simulink model "SensorFaultInj"  (R2013a)
settings: Solver=FixedStepDiscrete  SolverMode=SingleTasking  StartTime=0.0  StopTime=SimLength  FixedStep=SampleTime  RelTol=1e-3
values from neighbouring files (symbols this model uses):
  GlobalSeed = 10    [start_framework07.m]
  SampleTime = 0.01    [start_framework07.m]
  SimLength = 40    [start_framework07.m]
undefined symbols (not defined in the file or in its folder): DiscIntNeverNeededParam
libraries: dspswit3 x48, simulink x32
(part 6 of 9)

== system SensorFaultInj/FIM_Muster2/Parser Modul/schedule once per sample step /schedule_fcn id 6 ==
  In1 : Inport
  Discrete-Time Integrator : DiscreteIntegrator  SampleTime=-1  ICPrevOutput=DiscIntNeverNeededParam  ICPrevScaledInput=DiscIntNeverNeededParam
  Scope1 : Scope  NumInputPorts=2
      settings: YMin=-5~-5  YMax=5~5  SaveName=ScopeData25
  SimLength : Constant  Value=SimLength
  ex_sfun_schedulefcn1 : S-Function  FunctionName=ex_sfun_schedulefcn  EnableBusSupport=off  mask(Legacy Function){SFunctionSpec=single y1 = schedule_fcn(double u1, double u2, single u3, single u4), ShowSpec=on}
      mask prompts: ShowSpec "Display function specification"
      mask help:
      | This block allows you to call the legacy functions specified by the following Legacy Code Tool definition:
      | def.SFunctionName = 'ex_sfun_schedulefcn';
      | def.OutputFcnSpec = 'single y1 = schedule_fcn(double u1, double u2, single u3, single u4)';
      | def.HeaderFiles = {'schedule_fcn.hpp'};
      | def.SourceFiles = {'schedule_fcn.cpp'};
      | def.Options.language = 'C++';
      mask Help: <p>This block was generated automatically by the Legacy Code Tool. For detailed help on this tool, call<a href="matlab:legacy_code('help')"> legacy_code('help')</a>.</p>
      mask Callback ShowSpec:
      | if strcmp(get_param(gcbh, 'ShowSpec'), 'on')
      |   set_param(gcbh, 'MaskDisplay', sprintf('fprintf(''%s'');', get_param(gcbh, 'SFunctionSpec')));
      | else
      |   set_param(gcbh, 'MaskDisplay', sprintf('fprintf(''%s'');', get_param(gcbh, 'FunctionName')));
      | end
      mask Display: fprintf('single y1 = schedule_fcn(double u1, double u2, single u3, single u4)');
  "fault_id " : Constant  Value=6  OutDataTypeStr=single
  one : Constant
  output : Outport  OutputWhenDisabled=reset  InitialOutput=[0]
  wires:
  one/1 -> Discrete-Time Integrator/1
  Discrete-Time Integrator/1 -> ex_sfun_schedulefcn1/2, Scope1/2
  ex_sfun_schedulefcn1/1 -> Scope1/1, output/1  "out_schedule"
  SimLength/1 -> ex_sfun_schedulefcn1/1
  "fault_id "/1 -> ex_sfun_schedulefcn1/3
  In1/1 -> ex_sfun_schedulefcn1/4

== system SensorFaultInj/FIM_Muster2/Parser Modul/schedule once per sample step /schedule_fcn id 7 ==
  In1 : Inport
  Discrete-Time Integrator : DiscreteIntegrator  SampleTime=-1  ICPrevOutput=DiscIntNeverNeededParam  ICPrevScaledInput=DiscIntNeverNeededParam
  Scope1 : Scope  NumInputPorts=2
      settings: YMin=-5~-5  YMax=5~5  SaveName=ScopeData25
  SimLength : Constant  Value=SimLength
  ex_sfun_schedulefcn1 : S-Function  FunctionName=ex_sfun_schedulefcn  EnableBusSupport=off  mask(Legacy Function){SFunctionSpec=single y1 = schedule_fcn(double u1, double u2, single u3, single u4), ShowSpec=on}
      mask prompts: ShowSpec "Display function specification"
      mask help:
      | This block allows you to call the legacy functions specified by the following Legacy Code Tool definition:
      | def.SFunctionName = 'ex_sfun_schedulefcn';
      | def.OutputFcnSpec = 'single y1 = schedule_fcn(double u1, double u2, single u3, single u4)';
      | def.HeaderFiles = {'schedule_fcn.hpp'};
      | def.SourceFiles = {'schedule_fcn.cpp'};
      | def.Options.language = 'C++';
      mask Help: <p>This block was generated automatically by the Legacy Code Tool. For detailed help on this tool, call<a href="matlab:legacy_code('help')"> legacy_code('help')</a>.</p>
      mask Callback ShowSpec:
      | if strcmp(get_param(gcbh, 'ShowSpec'), 'on')
      |   set_param(gcbh, 'MaskDisplay', sprintf('fprintf(''%s'');', get_param(gcbh, 'SFunctionSpec')));
      | else
      |   set_param(gcbh, 'MaskDisplay', sprintf('fprintf(''%s'');', get_param(gcbh, 'FunctionName')));
      | end
      mask Display: fprintf('single y1 = schedule_fcn(double u1, double u2, single u3, single u4)');
  "fault_id " : Constant  Value=7  OutDataTypeStr=single
  one : Constant
  output : Outport  OutputWhenDisabled=reset  InitialOutput=[0]
  wires:
  one/1 -> Discrete-Time Integrator/1
  Discrete-Time Integrator/1 -> ex_sfun_schedulefcn1/2, Scope1/2
  ex_sfun_schedulefcn1/1 -> Scope1/1, output/1  "spi_schedule"
  SimLength/1 -> ex_sfun_schedulefcn1/1
  "fault_id "/1 -> ex_sfun_schedulefcn1/3
  In1/1 -> ex_sfun_schedulefcn1/4

== system SensorFaultInj/FIM_Muster2/Parser Modul/schedule once per sample step /schedule_fcn id 8 ==
  In1 : Inport
  Discrete-Time Integrator : DiscreteIntegrator  SampleTime=-1  ICPrevOutput=DiscIntNeverNeededParam  ICPrevScaledInput=DiscIntNeverNeededParam
  Scope1 : Scope  NumInputPorts=2
      settings: YMin=-5~-5  YMax=5~5  SaveName=ScopeData25
  SimLength : Constant  Value=SimLength
  ex_sfun_schedulefcn1 : S-Function  FunctionName=ex_sfun_schedulefcn  EnableBusSupport=off  mask(Legacy Function){SFunctionSpec=single y1 = schedule_fcn(double u1, double u2, single u3, single u4), ShowSpec=on}
      mask prompts: ShowSpec "Display function specification"
      mask help:
      | This block allows you to call the legacy functions specified by the following Legacy Code Tool definition:
      | def.SFunctionName = 'ex_sfun_schedulefcn';
      | def.OutputFcnSpec = 'single y1 = schedule_fcn(double u1, double u2, single u3, single u4)';
      | def.HeaderFiles = {'schedule_fcn.hpp'};
      | def.SourceFiles = {'schedule_fcn.cpp'};
      | def.Options.language = 'C++';
      mask Help: <p>This block was generated automatically by the Legacy Code Tool. For detailed help on this tool, call<a href="matlab:legacy_code('help')"> legacy_code('help')</a>.</p>
      mask Callback ShowSpec:
      | if strcmp(get_param(gcbh, 'ShowSpec'), 'on')
      |   set_param(gcbh, 'MaskDisplay', sprintf('fprintf(''%s'');', get_param(gcbh, 'SFunctionSpec')));
      | else
      |   set_param(gcbh, 'MaskDisplay', sprintf('fprintf(''%s'');', get_param(gcbh, 'FunctionName')));
      | end
      mask Display: fprintf('single y1 = schedule_fcn(double u1, double u2, single u3, single u4)');
  "fault_id " : Constant  Value=8  OutDataTypeStr=single
  one : Constant
  output : Outport  OutputWhenDisabled=reset  InitialOutput=[0]
  wires:
  one/1 -> Discrete-Time Integrator/1
  Discrete-Time Integrator/1 -> ex_sfun_schedulefcn1/2, Scope1/2
  ex_sfun_schedulefcn1/1 -> Scope1/1, output/1  "stz_schedule"
  SimLength/1 -> ex_sfun_schedulefcn1/1
  "fault_id "/1 -> ex_sfun_schedulefcn1/3
  In1/1 -> ex_sfun_schedulefcn1/4

== system SensorFaultInj/FIM_Muster2/Parser Modul/schedule once per sample step /schedule_fcn id 9 ==
  In1 : Inport
  Discrete-Time Integrator : DiscreteIntegrator  SampleTime=-1  ICPrevOutput=DiscIntNeverNeededParam  ICPrevScaledInput=DiscIntNeverNeededParam
  Scope1 : Scope  NumInputPorts=2
      settings: YMin=-5~-5  YMax=5~5  SaveName=ScopeData25
  SimLength : Constant  Value=SimLength
  ex_sfun_schedulefcn1 : S-Function  FunctionName=ex_sfun_schedulefcn  EnableBusSupport=off  mask(Legacy Function){SFunctionSpec=single y1 = schedule_fcn(double u1, double u2, single u3, single u4), ShowSpec=on}
      mask prompts: ShowSpec "Display function specification"
      mask help:
      | This block allows you to call the legacy functions specified by the following Legacy Code Tool definition:
      | def.SFunctionName = 'ex_sfun_schedulefcn';
      | def.OutputFcnSpec = 'single y1 = schedule_fcn(double u1, double u2, single u3, single u4)';
      | def.HeaderFiles = {'schedule_fcn.hpp'};
      | def.SourceFiles = {'schedule_fcn.cpp'};
      | def.Options.language = 'C++';
      mask Help: <p>This block was generated automatically by the Legacy Code Tool. For detailed help on this tool, call<a href="matlab:legacy_code('help')"> legacy_code('help')</a>.</p>
      mask Callback ShowSpec:
      | if strcmp(get_param(gcbh, 'ShowSpec'), 'on')
      |   set_param(gcbh, 'MaskDisplay', sprintf('fprintf(''%s'');', get_param(gcbh, 'SFunctionSpec')));
      | else
      |   set_param(gcbh, 'MaskDisplay', sprintf('fprintf(''%s'');', get_param(gcbh, 'FunctionName')));
      | end
      mask Display: fprintf('single y1 = schedule_fcn(double u1, double u2, single u3, single u4)');
  "fault_id " : Constant  Value=9  OutDataTypeStr=single
  one : Constant
  output : Outport  OutputWhenDisabled=reset  InitialOutput=[0]
  wires:
  one/1 -> Discrete-Time Integrator/1
  Discrete-Time Integrator/1 -> ex_sfun_schedulefcn1/2, Scope1/2
  ex_sfun_schedulefcn1/1 -> Scope1/1, output/1  "stx_schedule"
  SimLength/1 -> ex_sfun_schedulefcn1/1
  "fault_id "/1 -> ex_sfun_schedulefcn1/3
  In1/1 -> ex_sfun_schedulefcn1/4

== system SensorFaultInj/FIM_Muster/Fault Injection Modul/AFI - additive faults injection/non correated noise/pdf_parser ==
  xml id : Inport
  Constant : Constant
  Interpreted MATLAB Function : MATLABFcn  MATLABFcn=rand
  Scope : Scope  NumInputPorts=2
      settings: YMin=0~2.77556e-17  YMax=1~1  SaveName=ScopeData26  MaxDataPoints=50000
  ex_sfun_parsdistr : S-Function  FunctionName=ex_sfun_parsdistr  EnableBusSupport=off  mask(Legacy Function){SFunctionSpec=double y1 = pars_distr(single u1, single u2, double u3), ShowSpec=on}
      mask prompts: ShowSpec "Display function specification"
      mask help:
      | This block allows you to call the legacy functions specified by the following Legacy Code Tool definition:
      | def.SFunctionName = 'ex_sfun_parsdistr';
      | def.OutputFcnSpec = 'double y1 = pars_distr(single u1, single u2, double u3)';
      | def.HeaderFiles = {'pars_distr.hpp'};
      | def.SourceFiles = {'pars_distr.cpp'};
      | def.Options.language = 'C++';
      mask Help: <p>This block was generated automatically by the Legacy Code Tool. For detailed help on this tool, call<a href="matlab:legacy_code('help')"> legacy_code('help')</a>.</p>
      mask Callback ShowSpec:
      | if strcmp(get_param(gcbh, 'ShowSpec'), 'on')
      |   set_param(gcbh, 'MaskDisplay', sprintf('fprintf(''%s'');', get_param(gcbh, 'SFunctionSpec')));
      | else
      |   set_param(gcbh, 'MaskDisplay', sprintf('fprintf(''%s'');', get_param(gcbh, 'FunctionName')));
      | end
      mask Display: fprintf('double y1 = pars_distr(single u1, single u2, double u3)');
  "fault_id " : Constant  Value=5  OutDataTypeStr=single
  distr value : Outport
  wires:
  "fault_id "/1 -> ex_sfun_parsdistr/1
  xml id/1 -> ex_sfun_parsdistr/2
  ex_sfun_parsdistr/1 -> Scope/1, distr value/1
  Constant/1 -> Interpreted MATLAB Function/1
  Interpreted MATLAB Function/1 -> ex_sfun_parsdistr/3, Scope/2

== system SensorFaultInj/FIM_Muster/Fault Injection Modul/AFI - additive faults injection/stuck at x generation/Triggered Subsystem1 ==
  "In1 " : Inport
  Trigger : TriggerPort  TriggerType=either  PortDimensions=1
  Out1 : Outport
  wires:
  "In1 "/1 -> Out1/1

== system SensorFaultInj/FIM_Muster/Fault Injection Modul/AFI - additive faults injection/stuck at x generation1/Triggered Subsystem ==
  top border : Inport
  bottom border : Inport  Port=2
  Trigger : TriggerPort  TriggerType=either  PortDimensions=1
  Add1 : Sum
  Product2 : Product
  Scope : Scope
      settings: YMin=3  YMax=13  SaveName=ScopeData5
  Subtract : Sum  Inputs=+-
  Uniform Random Number : UniformRandomNumber  Minimum=0
  Out1 : Outport
  wires:
  Uniform Random Number/1 -> Product2/2
  top border/1 -> Subtract/1
  Subtract/1 -> Product2/1
  Product2/1 -> Add1/1
  Add1/1 -> Out1/1, Scope/1
  bottom border/1 -> Add1/2, Subtract/2

== system SensorFaultInj/FIM_Muster/Fault Injection Modul/FFI - functional fault injection/time correlated delay /expr_parser ==
  xml id : Inport
  Discrete-Time Integrator : DiscreteIntegrator  SampleTime=-1  ICPrevOutput=DiscIntNeverNeededParam  ICPrevScaledInput=DiscIntNeverNeededParam
  SampleTime : Constant  Value=SampleTime
  Scope1 : Scope  NumInputPorts=2
      settings: YMin=-5~-5  YMax=5~5  SaveName=ScopeData24
  SimLength : Constant  Value=SimLength
  ex_sfun_parsfcn : S-Function  FunctionName=ex_sfun_parsfcn  EnableBusSupport=off  mask(Legacy Function){SFunctionSpec=double y1 = pars_fcn(double u1, double u2, double u3, double u4, single u5), ShowSpec=on}
      mask prompts: ShowSpec "Display function specification"
      mask help:
      | This block allows you to call the legacy functions specified by the following Legacy Code Tool definition:
      | def.SFunctionName = 'ex_sfun_parsfcn';
      | def.OutputFcnSpec = 'double y1 = pars_fcn(double u1, double u2, double u3, double u4, single u5)';
      | def.HeaderFiles = {'pars_fcn.hpp'};
      | def.SourceFiles = {'pars_fcn.cpp'};
      | def.Options.language = 'C++';
      mask Help: <p>This block was generated automatically by the Legacy Code Tool. For detailed help on this tool, call<a href="matlab:legacy_code('help')"> legacy_code('help')</a>.</p>
      mask Callback ShowSpec:
      | if strcmp(get_param(gcbh, 'ShowSpec'), 'on')
      |   set_param(gcbh, 'MaskDisplay', sprintf('fprintf(''%s'');', get_param(gcbh, 'SFunctionSpec')));
      | else
      |   set_param(gcbh, 'MaskDisplay', sprintf('fprintf(''%s'');', get_param(gcbh, 'FunctionName')));
      | end
      mask Display: fprintf('double y1 = pars_fcn(double u1, double u2, double u3, double u4, single u5)');
  "fault_id " : Constant  Value=3
  one : Constant
  corelation value : Outport
  wires:
  one/1 -> Discrete-Time Integrator/1
  Discrete-Time Integrator/1 -> ex_sfun_parsfcn/4, Scope1/2
  "fault_id "/1 -> ex_sfun_parsfcn/1
  SampleTime/1 -> ex_sfun_parsfcn/2
  SimLength/1 -> ex_sfun_parsfcn/3
  xml id/1 -> ex_sfun_parsfcn/5
  ex_sfun_parsfcn/1 -> Scope1/1, corelation value/1

== system SensorFaultInj/FIM_Muster/Fault Injection Modul/MFI - multiplicative fault injection/time correlated noise/expr_parser1 ==
  xml id : Inport
  Discrete-Time Integrator : DiscreteIntegrator  SampleTime=-1  ICPrevOutput=DiscIntNeverNeededParam  ICPrevScaledInput=DiscIntNeverNeededParam
  SampleTime : Constant  Value=SampleTime
  Scope1 : Scope  NumInputPorts=2
      settings: YMin=-5~-5  YMax=5~5  SaveName=ScopeData24
  SimLength : Constant  Value=SimLength
  ex_sfun_parsfcn : S-Function  FunctionName=ex_sfun_parsfcn  EnableBusSupport=off  mask(Legacy Function){SFunctionSpec=double y1 = pars_fcn(double u1, double u2, double u3, double u4, single u5), ShowSpec=on}
      mask prompts: ShowSpec "Display function specification"
      mask help:
      | This block allows you to call the legacy functions specified by the following Legacy Code Tool definition:
      | def.SFunctionName = 'ex_sfun_parsfcn';
      | def.OutputFcnSpec = 'double y1 = pars_fcn(double u1, double u2, double u3, double u4, single u5)';
      | def.HeaderFiles = {'pars_fcn.hpp'};
      | def.SourceFiles = {'pars_fcn.cpp'};
      | def.Options.language = 'C++';
      mask Help: <p>This block was generated automatically by the Legacy Code Tool. For detailed help on this tool, call<a href="matlab:legacy_code('help')"> legacy_code('help')</a>.</p>
      mask Callback ShowSpec:
      | if strcmp(get_param(gcbh, 'ShowSpec'), 'on')
      |   set_param(gcbh, 'MaskDisplay', sprintf('fprintf(''%s'');', get_param(gcbh, 'SFunctionSpec')));
      | else
      |   set_param(gcbh, 'MaskDisplay', sprintf('fprintf(''%s'');', get_param(gcbh, 'FunctionName')));
      | end
      mask Display: fprintf('double y1 = pars_fcn(double u1, double u2, double u3, double u4, single u5)');
  "fault_id " : Constant  Value=2
  one : Constant
  corelation value : Outport
  wires:
  one/1 -> Discrete-Time Integrator/1
  Discrete-Time Integrator/1 -> ex_sfun_parsfcn/4, Scope1/2
  "fault_id "/1 -> ex_sfun_parsfcn/1
  SampleTime/1 -> ex_sfun_parsfcn/2
  SimLength/1 -> ex_sfun_parsfcn/3
  xml id/1 -> ex_sfun_parsfcn/5
  ex_sfun_parsfcn/1 -> Scope1/1, corelation value/1

== system SensorFaultInj/FIM_Muster/Fault Injection Modul/MFI - multiplicative fault injection/time correlated noise/pdf_parser ==
  xml id : Inport
  Constant : Constant
  Interpreted MATLAB Function : MATLABFcn  MATLABFcn=rand
  Scope : Scope  NumInputPorts=2
      settings: YMin=0.05~2.77556e-17  YMax=0.85~1  SaveName=ScopeData26  MaxDataPoints=50000
  ex_sfun_parsdistr : S-Function  FunctionName=ex_sfun_parsdistr  EnableBusSupport=off  mask(Legacy Function){SFunctionSpec=double y1 = pars_distr(single u1, single u2, double u3), ShowSpec=on}
      mask prompts: ShowSpec "Display function specification"
      mask help:
      | This block allows you to call the legacy functions specified by the following Legacy Code Tool definition:
      | def.SFunctionName = 'ex_sfun_parsdistr';
      | def.OutputFcnSpec = 'double y1 = pars_distr(single u1, single u2, double u3)';
      | def.HeaderFiles = {'pars_distr.hpp'};
      | def.SourceFiles = {'pars_distr.cpp'};
      | def.Options.language = 'C++';
      mask Help: <p>This block was generated automatically by the Legacy Code Tool. For detailed help on this tool, call<a href="matlab:legacy_code('help')"> legacy_code('help')</a>.</p>
      mask Callback ShowSpec:
      | if strcmp(get_param(gcbh, 'ShowSpec'), 'on')
      |   set_param(gcbh, 'MaskDisplay', sprintf('fprintf(''%s'');', get_param(gcbh, 'SFunctionSpec')));
      | else
      |   set_param(gcbh, 'MaskDisplay', sprintf('fprintf(''%s'');', get_param(gcbh, 'FunctionName')));
      | end
      mask Display: fprintf('double y1 = pars_distr(single u1, single u2, double u3)');
  "fault_id " : Constant  Value=3  OutDataTypeStr=single
  distr value : Outport
  wires:
  "fault_id "/1 -> ex_sfun_parsdistr/1
  xml id/1 -> ex_sfun_parsdistr/2
  ex_sfun_parsdistr/1 -> Scope/1, distr value/1
  Constant/1 -> Interpreted MATLAB Function/1
  Interpreted MATLAB Function/1 -> ex_sfun_parsdistr/3, Scope/2

== system SensorFaultInj/FIM_Muster/Fault Injection Modul/MFI - multiplicative fault injection/time correlated offset/expr_parser ==
  xml id : Inport
  Discrete-Time Integrator : DiscreteIntegrator  SampleTime=-1  ICPrevOutput=DiscIntNeverNeededParam  ICPrevScaledInput=DiscIntNeverNeededParam
  SampleTime : Constant  Value=SampleTime
  Scope1 : Scope  NumInputPorts=2
      settings: YMin=-5~-5  YMax=5~5  SaveName=ScopeData24
  SimLength : Constant  Value=SimLength
  ex_sfun_parsfcn : S-Function  FunctionName=ex_sfun_parsfcn  EnableBusSupport=off  mask(Legacy Function){SFunctionSpec=double y1 = pars_fcn(double u1, double u2, double u3, double u4, single u5), ShowSpec=on}
      mask prompts: ShowSpec "Display function specification"
      mask help:
      | This block allows you to call the legacy functions specified by the following Legacy Code Tool definition:
      | def.SFunctionName = 'ex_sfun_parsfcn';
      | def.OutputFcnSpec = 'double y1 = pars_fcn(double u1, double u2, double u3, double u4, single u5)';
      | def.HeaderFiles = {'pars_fcn.hpp'};
      | def.SourceFiles = {'pars_fcn.cpp'};
      | def.Options.language = 'C++';
      mask Help: <p>This block was generated automatically by the Legacy Code Tool. For detailed help on this tool, call<a href="matlab:legacy_code('help')"> legacy_code('help')</a>.</p>
      mask Callback ShowSpec:
      | if strcmp(get_param(gcbh, 'ShowSpec'), 'on')
      |   set_param(gcbh, 'MaskDisplay', sprintf('fprintf(''%s'');', get_param(gcbh, 'SFunctionSpec')));
      | else
      |   set_param(gcbh, 'MaskDisplay', sprintf('fprintf(''%s'');', get_param(gcbh, 'FunctionName')));
      | end
      mask Display: fprintf('double y1 = pars_fcn(double u1, double u2, double u3, double u4, single u5)');
  "fault_id " : Constant
  one : Constant
  corelation value : Outport
  wires:
  one/1 -> Discrete-Time Integrator/1
  Discrete-Time Integrator/1 -> ex_sfun_parsfcn/4, Scope1/2
  "fault_id "/1 -> ex_sfun_parsfcn/1
  SampleTime/1 -> ex_sfun_parsfcn/2
  SimLength/1 -> ex_sfun_parsfcn/3
  xml id/1 -> ex_sfun_parsfcn/5
  ex_sfun_parsfcn/1 -> Scope1/1, corelation value/1

== system SensorFaultInj/FIM_Muster/Fault Injection Modul/MFI - multiplicative fault injection/value correlated noise/pdf_parser ==
  xml id : Inport
  Constant : Constant
  Interpreted MATLAB Function : MATLABFcn  MATLABFcn=rand
  Scope : Scope  NumInputPorts=2
      settings: YMin=0.05~2.77556e-17  YMax=0.85~1  SaveName=ScopeData26  MaxDataPoints=50000
  ex_sfun_parsdistr : S-Function  FunctionName=ex_sfun_parsdistr  EnableBusSupport=off  mask(Legacy Function){SFunctionSpec=double y1 = pars_distr(single u1, single u2, double u3), ShowSpec=on}
      mask prompts: ShowSpec "Display function specification"
      mask help:
      | This block allows you to call the legacy functions specified by the following Legacy Code Tool definition:
      | def.SFunctionName = 'ex_sfun_parsdistr';
      | def.OutputFcnSpec = 'double y1 = pars_distr(single u1, single u2, double u3)';
      | def.HeaderFiles = {'pars_distr.hpp'};
      | def.SourceFiles = {'pars_distr.cpp'};
      | def.Options.language = 'C++';
      mask Help: <p>This block was generated automatically by the Legacy Code Tool. For detailed help on this tool, call<a href="matlab:legacy_code('help')"> legacy_code('help')</a>.</p>
      mask Callback ShowSpec:
      | if strcmp(get_param(gcbh, 'ShowSpec'), 'on')
      |   set_param(gcbh, 'MaskDisplay', sprintf('fprintf(''%s'');', get_param(gcbh, 'SFunctionSpec')));
      | else
      |   set_param(gcbh, 'MaskDisplay', sprintf('fprintf(''%s'');', get_param(gcbh, 'FunctionName')));
      | end
      mask Display: fprintf('double y1 = pars_distr(single u1, single u2, double u3)');
  "fault_id " : Constant  Value=2  OutDataTypeStr=single
  distr value : Outport
  wires:
  "fault_id "/1 -> ex_sfun_parsdistr/1
  xml id/1 -> ex_sfun_parsdistr/2
  ex_sfun_parsdistr/1 -> Scope/1, distr value/1
  Constant/1 -> Interpreted MATLAB Function/1
  Interpreted MATLAB Function/1 -> ex_sfun_parsdistr/3, Scope/2

== system SensorFaultInj/FIM_Muster/Parser Modul/Fault Parameter Parser/Enabled Subsystem/param_fcn id 0 ==
  In1 : Inport
  parser_fcn param id 2 : Subsystem
  Out1 : Outport
  wires:
  parser_fcn param id 2/1(output) -> Out1/1  "vco_factor"
  In1/1 -> parser_fcn param id 2/1(input)

== system SensorFaultInj/FIM_Muster/Parser Modul/Fault Parameter Parser/Enabled Subsystem/param_fcn id 1 ==
  In1 : Inport
  parser_fcn param id 2 : Subsystem
  Out1 : Outport
  wires:
  parser_fcn param id 2/1(output) -> Out1/1  "tco_amplitude"
  In1/1 -> parser_fcn param id 2/1(input)

== system SensorFaultInj/FIM_Muster/Parser Modul/Fault Parameter Parser/Enabled Subsystem/param_fcn id 10 ==
  In1 : Inport
  Bus Creator : BusCreator  Inputs=2
  parser_fcn param id 0 : Subsystem
  parser_fcn param id 1 : Subsystem
  Out1 : Outport
  wires:
  parser_fcn param id 0/1(output) -> Bus Creator/1  "sat_top"
  parser_fcn param id 1/1(output) -> Bus Creator/2  "sat_bot"
  Bus Creator/1 -> Out1/1  "sat_param_bus"
  In1/1 -> parser_fcn param id 0/1(input), parser_fcn param id 1/1(input)

== system SensorFaultInj/FIM_Muster/Parser Modul/Fault Parameter Parser/Enabled Subsystem/param_fcn id 11 ==
  In1 : Inport
  parser_fcn param id 2 : Subsystem
  Out1 : Outport
  wires:
  parser_fcn param id 2/1(output) -> Out1/1  "ncd_delay"
  In1/1 -> parser_fcn param id 2/1(input)

== system SensorFaultInj/FIM_Muster/Parser Modul/Fault Parameter Parser/Enabled Subsystem/param_fcn id 12 ==
  In1 : Inport
  parser_fcn param id 2 : Subsystem
  Out1 : Outport
  wires:
  parser_fcn param id 2/1(output) -> Out1/1  "tcd_delay"
  In1/1 -> parser_fcn param id 2/1(input)

== system SensorFaultInj/FIM_Muster/Parser Modul/Fault Parameter Parser/Enabled Subsystem/param_fcn id 2 ==
  In1 : Inport
  parser_fcn param id 3 : Subsystem
  Out1 : Outport
  wires:
  In1/1 -> parser_fcn param id 3/1(input)
  parser_fcn param id 3/1(output) -> Out1/1  "vcn_factor"

== system SensorFaultInj/FIM_Muster/Parser Modul/Fault Parameter Parser/Enabled Subsystem/param_fcn id 3 ==
  In1 : Inport
  parser_fcn param id 2 : Subsystem
  Out1 : Outport
  wires:
  parser_fcn param id 2/1(output) -> Out1/1  "tcn_factor"
  In1/1 -> parser_fcn param id 2/1(input)

== system SensorFaultInj/FIM_Muster/Parser Modul/Fault Parameter Parser/Enabled Subsystem/param_fcn id 4 ==
  In1 : Inport
  parser_fcn param id 2 : Subsystem
  Out1 : Outport
  wires:
  parser_fcn param id 2/1(output) -> Out1/1  "nco_amplitude"
  In1/1 -> parser_fcn param id 2/1(input)

== system SensorFaultInj/FIM_Muster/Parser Modul/Fault Parameter Parser/Enabled Subsystem/param_fcn id 5 ==
  In1 : Inport
  parser_fcn param id 2 : Subsystem
  Out1 : Outport
  wires:
  parser_fcn param id 2/1(output) -> Out1/1  "ncn_factor"
  In1/1 -> parser_fcn param id 2/1(input)

== system SensorFaultInj/FIM_Muster/Parser Modul/Fault Parameter Parser/Enabled Subsystem/param_fcn id 6 ==
  In1 : Inport
  Bus Creator : BusCreator  Inputs=2
  parser_fcn param id 2 : Subsystem
  parser_fcn param id 3 : Subsystem
  Out1 : Outport
  wires:
  parser_fcn param id 2/1(output) -> Bus Creator/1  "out_amplitude"
  parser_fcn param id 3/1(output) -> Bus Creator/2  "out_neg"
  Bus Creator/1 -> Out1/1  "out_param_bus"
  In1/1 -> parser_fcn param id 2/1(input), parser_fcn param id 3/1(input)

== system SensorFaultInj/FIM_Muster/Parser Modul/Fault Parameter Parser/Enabled Subsystem/param_fcn id 7 ==
  In1 : Inport
  Bus Creator : BusCreator  Inputs=2
  parser_fcn param id 0 : Subsystem
  parser_fcn param id 1 : Subsystem
  Out1 : Outport
  wires:
  parser_fcn param id 1/1(output) -> Bus Creator/2  "spi_length"
  parser_fcn param id 0/1(output) -> Bus Creator/1  "spi_factor"
  Bus Creator/1 -> Out1/1  "spi_param_bus"
  In1/1 -> parser_fcn param id 1/1(input), parser_fcn param id 0/1(input)

== system SensorFaultInj/FIM_Muster/Parser Modul/Fault Parameter Parser/Enabled Subsystem/param_fcn id 8 ==
  In1 : Inport
  parser_fcn param id 0 : Subsystem
  Out1 : Outport
  wires:
  parser_fcn param id 0/1(output) -> Out1/1  "stz_length"
  In1/1 -> parser_fcn param id 0/1(input)

== system SensorFaultInj/FIM_Muster/Parser Modul/Fault Parameter Parser/Enabled Subsystem/param_fcn id 9 ==
  In1 : Inport
  Bus Creator : BusCreator  Inputs=3
  parser_fcn param id 1 : Subsystem
  parser_fcn param id 2 : Subsystem
  parser_fcn param id 3 : Subsystem
  Out1 : Outport
  wires:
  parser_fcn param id 2/1(output) -> Bus Creator/1  "stx_max"
  parser_fcn param id 3/1(output) -> Bus Creator/2  "stx_min"
  Bus Creator/1 -> Out1/1  "stx_param_bus"
  In1/1 -> parser_fcn param id 1/1(input), parser_fcn param id 2/1(input), parser_fcn param id 3/1(input)
  parser_fcn param id 1/1(output) -> Bus Creator/3  "stx_length"

== system SensorFaultInj/FIM_Muster/Parser Modul/Occurence Parser /Enabled Subsystem/occurnce parser fault id 2 ==
  In1 : Inport
  ex_sfun_occfcn : S-Function  FunctionName=ex_sfun_occfcn  EnableBusSupport=off  mask(Legacy Function){SFunctionSpec=double y1 = occ_fcn(single u1, single u2), ShowSpec=on}
      mask prompts: ShowSpec "Display function specification"
      mask help:
      | This block allows you to call the legacy functions specified by the following Legacy Code Tool definition:
      | def.SFunctionName = 'ex_sfun_occfcn';
      | def.OutputFcnSpec = 'double y1 = occ_fcn(single u1, single u2)';
      | def.HeaderFiles = {'occ_fcn.hpp'};
      | def.SourceFiles = {'occ_fcn.cpp'};
      | def.Options.language = 'C++';
      mask Help: <p>This block was generated automatically by the Legacy Code Tool. For detailed help on this tool, call<a href="matlab:legacy_code('help')"> legacy_code('help')</a>.</p>
      mask Callback ShowSpec:
      | if strcmp(get_param(gcbh, 'ShowSpec'), 'on')
      |   set_param(gcbh, 'MaskDisplay', sprintf('fprintf(''%s'');', get_param(gcbh, 'SFunctionSpec')));
      | else
      |   set_param(gcbh, 'MaskDisplay', sprintf('fprintf(''%s'');', get_param(gcbh, 'FunctionName')));
      | end
      mask Display: fprintf('double y1 = occ_fcn(single u1, single u2)');
  "fault_id " : Constant  Value=2  OutDataTypeStr=single
  Out1 : Outport
  wires:
  ex_sfun_occfcn/1 -> Out1/1  "vcn_occ"
  "fault_id "/1 -> ex_sfun_occfcn/1
  In1/1 -> ex_sfun_occfcn/2

== system SensorFaultInj/FIM_Muster/Parser Modul/Occurence Parser /Enabled Subsystem/occurnce parser fault id 3 ==
  In1 : Inport
  ex_sfun_occfcn : S-Function  FunctionName=ex_sfun_occfcn  EnableBusSupport=off  mask(Legacy Function){SFunctionSpec=double y1 = occ_fcn(single u1, single u2), ShowSpec=on}
      mask prompts: ShowSpec "Display function specification"
      mask help:
      | This block allows you to call the legacy functions specified by the following Legacy Code Tool definition:
      | def.SFunctionName = 'ex_sfun_occfcn';
      | def.OutputFcnSpec = 'double y1 = occ_fcn(single u1, single u2)';
      | def.HeaderFiles = {'occ_fcn.hpp'};
      | def.SourceFiles = {'occ_fcn.cpp'};
      | def.Options.language = 'C++';
      mask Help: <p>This block was generated automatically by the Legacy Code Tool. For detailed help on this tool, call<a href="matlab:legacy_code('help')"> legacy_code('help')</a>.</p>
      mask Callback ShowSpec:
      | if strcmp(get_param(gcbh, 'ShowSpec'), 'on')
      |   set_param(gcbh, 'MaskDisplay', sprintf('fprintf(''%s'');', get_param(gcbh, 'SFunctionSpec')));
      | else
      |   set_param(gcbh, 'MaskDisplay', sprintf('fprintf(''%s'');', get_param(gcbh, 'FunctionName')));
      | end
      mask Display: fprintf('double y1 = occ_fcn(single u1, single u2)');
  "fault_id " : Constant  Value=3  OutDataTypeStr=single
  Out1 : Outport
  wires:
  "fault_id "/1 -> ex_sfun_occfcn/1
  ex_sfun_occfcn/1 -> Out1/1  "tcn_occ"
  In1/1 -> ex_sfun_occfcn/2

== system SensorFaultInj/FIM_Muster/Parser Modul/Occurence Parser /Enabled Subsystem/occurnce parser fault id 5 ==
  In1 : Inport
  ex_sfun_occfcn : S-Function  FunctionName=ex_sfun_occfcn  EnableBusSupport=off  mask(Legacy Function){SFunctionSpec=double y1 = occ_fcn(single u1, single u2), ShowSpec=on}
      mask prompts: ShowSpec "Display function specification"
      mask help:
      | This block allows you to call the legacy functions specified by the following Legacy Code Tool definition:
      | def.SFunctionName = 'ex_sfun_occfcn';
      | def.OutputFcnSpec = 'double y1 = occ_fcn(single u1, single u2)';
      | def.HeaderFiles = {'occ_fcn.hpp'};
      | def.SourceFiles = {'occ_fcn.cpp'};
      | def.Options.language = 'C++';
      mask Help: <p>This block was generated automatically by the Legacy Code Tool. For detailed help on this tool, call<a href="matlab:legacy_code('help')"> legacy_code('help')</a>.</p>
      mask Callback ShowSpec:
      | if strcmp(get_param(gcbh, 'ShowSpec'), 'on')
      |   set_param(gcbh, 'MaskDisplay', sprintf('fprintf(''%s'');', get_param(gcbh, 'SFunctionSpec')));
      | else
      |   set_param(gcbh, 'MaskDisplay', sprintf('fprintf(''%s'');', get_param(gcbh, 'FunctionName')));
      | end
      mask Display: fprintf('double y1 = occ_fcn(single u1, single u2)');
  "fault_id " : Constant  Value=5  OutDataTypeStr=single
  Out1 : Outport
  wires:
  "fault_id "/1 -> ex_sfun_occfcn/1
  ex_sfun_occfcn/1 -> Out1/1  "ncn_occ"
  In1/1 -> ex_sfun_occfcn/2

== system SensorFaultInj/FIM_Muster/Parser Modul/Occurence Parser /Enabled Subsystem/occurnce parser fault id 6 ==
  In1 : Inport
  ex_sfun_occfcn : S-Function  FunctionName=ex_sfun_occfcn  EnableBusSupport=off  mask(Legacy Function){SFunctionSpec=double y1 = occ_fcn(single u1, single u2), ShowSpec=on}
      mask prompts: ShowSpec "Display function specification"
      mask help:
      | This block allows you to call the legacy functions specified by the following Legacy Code Tool definition:
      | def.SFunctionName = 'ex_sfun_occfcn';
      | def.OutputFcnSpec = 'double y1 = occ_fcn(single u1, single u2)';
      | def.HeaderFiles = {'occ_fcn.hpp'};
      | def.SourceFiles = {'occ_fcn.cpp'};
      | def.Options.language = 'C++';
      mask Help: <p>This block was generated automatically by the Legacy Code Tool. For detailed help on this tool, call<a href="matlab:legacy_code('help')"> legacy_code('help')</a>.</p>
      mask Callback ShowSpec:
      | if strcmp(get_param(gcbh, 'ShowSpec'), 'on')
      |   set_param(gcbh, 'MaskDisplay', sprintf('fprintf(''%s'');', get_param(gcbh, 'SFunctionSpec')));
      | else
      |   set_param(gcbh, 'MaskDisplay', sprintf('fprintf(''%s'');', get_param(gcbh, 'FunctionName')));
      | end
      mask Display: fprintf('double y1 = occ_fcn(single u1, single u2)');
  "fault_id " : Constant  Value=6  OutDataTypeStr=single
  Out1 : Outport
  wires:
  "fault_id "/1 -> ex_sfun_occfcn/1
  ex_sfun_occfcn/1 -> Out1/1  "out_occ"
  In1/1 -> ex_sfun_occfcn/2

== system SensorFaultInj/FIM_Muster/Parser Modul/Occurence Parser /Enabled Subsystem/occurnce parser fault id 7 ==
  In1 : Inport
  ex_sfun_occfcn : S-Function  FunctionName=ex_sfun_occfcn  EnableBusSupport=off  mask(Legacy Function){SFunctionSpec=double y1 = occ_fcn(single u1, single u2), ShowSpec=on}
      mask prompts: ShowSpec "Display function specification"
      mask help:
      | This block allows you to call the legacy functions specified by the following Legacy Code Tool definition:
      | def.SFunctionName = 'ex_sfun_occfcn';
      | def.OutputFcnSpec = 'double y1 = occ_fcn(single u1, single u2)';
      | def.HeaderFiles = {'occ_fcn.hpp'};
      | def.SourceFiles = {'occ_fcn.cpp'};
      | def.Options.language = 'C++';
      mask Help: <p>This block was generated automatically by the Legacy Code Tool. For detailed help on this tool, call<a href="matlab:legacy_code('help')"> legacy_code('help')</a>.</p>
      mask Callback ShowSpec:
      | if strcmp(get_param(gcbh, 'ShowSpec'), 'on')
      |   set_param(gcbh, 'MaskDisplay', sprintf('fprintf(''%s'');', get_param(gcbh, 'SFunctionSpec')));
      | else
      |   set_param(gcbh, 'MaskDisplay', sprintf('fprintf(''%s'');', get_param(gcbh, 'FunctionName')));
      | end
      mask Display: fprintf('double y1 = occ_fcn(single u1, single u2)');
  "fault_id " : Constant  Value=7  OutDataTypeStr=single
  Out1 : Outport
  wires:
  "fault_id "/1 -> ex_sfun_occfcn/1
  ex_sfun_occfcn/1 -> Out1/1  "spi_occ"
  In1/1 -> ex_sfun_occfcn/2

== system SensorFaultInj/FIM_Muster/Parser Modul/Occurence Parser /Enabled Subsystem/occurnce parser fault id 8 ==
  In1 : Inport
  ex_sfun_occfcn : S-Function  FunctionName=ex_sfun_occfcn  EnableBusSupport=off  mask(Legacy Function){SFunctionSpec=double y1 = occ_fcn(single u1, single u2), ShowSpec=on}
      mask prompts: ShowSpec "Display function specification"
      mask help:
      | This block allows you to call the legacy functions specified by the following Legacy Code Tool definition:
      | def.SFunctionName = 'ex_sfun_occfcn';
      | def.OutputFcnSpec = 'double y1 = occ_fcn(single u1, single u2)';
      | def.HeaderFiles = {'occ_fcn.hpp'};
      | def.SourceFiles = {'occ_fcn.cpp'};
      | def.Options.language = 'C++';
      mask Help: <p>This block was generated automatically by the Legacy Code Tool. For detailed help on this tool, call<a href="matlab:legacy_code('help')"> legacy_code('help')</a>.</p>
      mask Callback ShowSpec:
      | if strcmp(get_param(gcbh, 'ShowSpec'), 'on')
      |   set_param(gcbh, 'MaskDisplay', sprintf('fprintf(''%s'');', get_param(gcbh, 'SFunctionSpec')));
      | else
      |   set_param(gcbh, 'MaskDisplay', sprintf('fprintf(''%s'');', get_param(gcbh, 'FunctionName')));
      | end
      mask Display: fprintf('double y1 = occ_fcn(single u1, single u2)');
  "fault_id " : Constant  Value=8  OutDataTypeStr=single
  Out1 : Outport
  wires:
  "fault_id "/1 -> ex_sfun_occfcn/1
  ex_sfun_occfcn/1 -> Out1/1  "stz_occ"
  In1/1 -> ex_sfun_occfcn/2

== system SensorFaultInj/FIM_Muster/Parser Modul/Occurence Parser /Enabled Subsystem/occurnce parser fault id 9 ==
  In1 : Inport
  ex_sfun_occfcn : S-Function  FunctionName=ex_sfun_occfcn  EnableBusSupport=off  mask(Legacy Function){SFunctionSpec=double y1 = occ_fcn(single u1, single u2), ShowSpec=on}
      mask prompts: ShowSpec "Display function specification"
      mask help:
      | This block allows you to call the legacy functions specified by the following Legacy Code Tool definition:
      | def.SFunctionName = 'ex_sfun_occfcn';
      | def.OutputFcnSpec = 'double y1 = occ_fcn(single u1, single u2)';
      | def.HeaderFiles = {'occ_fcn.hpp'};
      | def.SourceFiles = {'occ_fcn.cpp'};
      | def.Options.language = 'C++';
      mask Help: <p>This block was generated automatically by the Legacy Code Tool. For detailed help on this tool, call<a href="matlab:legacy_code('help')"> legacy_code('help')</a>.</p>
      mask Callback ShowSpec:
      | if strcmp(get_param(gcbh, 'ShowSpec'), 'on')
      |   set_param(gcbh, 'MaskDisplay', sprintf('fprintf(''%s'');', get_param(gcbh, 'SFunctionSpec')));
      | else
      |   set_param(gcbh, 'MaskDisplay', sprintf('fprintf(''%s'');', get_param(gcbh, 'FunctionName')));
      | end
      mask Display: fprintf('double y1 = occ_fcn(single u1, single u2)');
  "fault_id " : Constant  Value=9  OutDataTypeStr=single
  Out1 : Outport
  wires:
  "fault_id "/1 -> ex_sfun_occfcn/1
  ex_sfun_occfcn/1 -> Out1/1  "stx_occ"
  In1/1 -> ex_sfun_occfcn/2

== system SensorFaultInj/FIM_Muster1/Fault Injection Modul/AFI - additive faults injection/non correated noise/pdf_parser ==
  xml id : Inport
  Constant : Constant
  Interpreted MATLAB Function : MATLABFcn  MATLABFcn=rand
  Scope : Scope  NumInputPorts=2
      settings: YMin=0~2.77556e-17  YMax=1~1  SaveName=ScopeData26  MaxDataPoints=50000
  ex_sfun_parsdistr : S-Function  FunctionName=ex_sfun_parsdistr  EnableBusSupport=off  mask(Legacy Function){SFunctionSpec=double y1 = pars_distr(single u1, single u2, double u3), ShowSpec=on}
      mask prompts: ShowSpec "Display function specification"
      mask help:
      | This block allows you to call the legacy functions specified by the following Legacy Code Tool definition:
      | def.SFunctionName = 'ex_sfun_parsdistr';
      | def.OutputFcnSpec = 'double y1 = pars_distr(single u1, single u2, double u3)';
      | def.HeaderFiles = {'pars_distr.hpp'};
      | def.SourceFiles = {'pars_distr.cpp'};
      | def.Options.language = 'C++';
      mask Help: <p>This block was generated automatically by the Legacy Code Tool. For detailed help on this tool, call<a href="matlab:legacy_code('help')"> legacy_code('help')</a>.</p>
      mask Callback ShowSpec:
      | if strcmp(get_param(gcbh, 'ShowSpec'), 'on')
      |   set_param(gcbh, 'MaskDisplay', sprintf('fprintf(''%s'');', get_param(gcbh, 'SFunctionSpec')));
      | else
      |   set_param(gcbh, 'MaskDisplay', sprintf('fprintf(''%s'');', get_param(gcbh, 'FunctionName')));
      | end
      mask Display: fprintf('double y1 = pars_distr(single u1, single u2, double u3)');
  "fault_id " : Constant  Value=5  OutDataTypeStr=single
  distr value : Outport
  wires:
  "fault_id "/1 -> ex_sfun_parsdistr/1
  xml id/1 -> ex_sfun_parsdistr/2
  ex_sfun_parsdistr/1 -> Scope/1, distr value/1
  Constant/1 -> Interpreted MATLAB Function/1
  Interpreted MATLAB Function/1 -> ex_sfun_parsdistr/3, Scope/2

== system SensorFaultInj/FIM_Muster1/Fault Injection Modul/AFI - additive faults injection/stuck at x generation/Triggered Subsystem1 ==
  "In1 " : Inport
  Trigger : TriggerPort  TriggerType=either  PortDimensions=1
  Out1 : Outport
  wires:
  "In1 "/1 -> Out1/1

== system SensorFaultInj/FIM_Muster1/Fault Injection Modul/AFI - additive faults injection/stuck at x generation1/Triggered Subsystem ==
  top border : Inport
  bottom border : Inport  Port=2
  Trigger : TriggerPort  TriggerType=either  PortDimensions=1
  Add1 : Sum
  Product2 : Product
  Scope : Scope
      settings: YMin=3  YMax=13  SaveName=ScopeData5
  Subtract : Sum  Inputs=+-
  Uniform Random Number : UniformRandomNumber  Minimum=0
  Out1 : Outport
  wires:
  Uniform Random Number/1 -> Product2/2
  top border/1 -> Subtract/1
  Subtract/1 -> Product2/1
  Product2/1 -> Add1/1
  Add1/1 -> Out1/1, Scope/1
  bottom border/1 -> Add1/2, Subtract/2

== system SensorFaultInj/FIM_Muster1/Fault Injection Modul/FFI - functional fault injection/time correlated delay /expr_parser ==
  xml id : Inport
  Discrete-Time Integrator : DiscreteIntegrator  SampleTime=-1  ICPrevOutput=DiscIntNeverNeededParam  ICPrevScaledInput=DiscIntNeverNeededParam
  SampleTime : Constant  Value=SampleTime
  Scope1 : Scope  NumInputPorts=2
      settings: YMin=-5~-5  YMax=5~5  SaveName=ScopeData24
  SimLength : Constant  Value=SimLength
  ex_sfun_parsfcn : S-Function  FunctionName=ex_sfun_parsfcn  EnableBusSupport=off  mask(Legacy Function){SFunctionSpec=double y1 = pars_fcn(double u1, double u2, double u3, double u4, single u5), ShowSpec=on}
      mask prompts: ShowSpec "Display function specification"
      mask help:
      | This block allows you to call the legacy functions specified by the following Legacy Code Tool definition:
      | def.SFunctionName = 'ex_sfun_parsfcn';
      | def.OutputFcnSpec = 'double y1 = pars_fcn(double u1, double u2, double u3, double u4, single u5)';
      | def.HeaderFiles = {'pars_fcn.hpp'};
      | def.SourceFiles = {'pars_fcn.cpp'};
      | def.Options.language = 'C++';
      mask Help: <p>This block was generated automatically by the Legacy Code Tool. For detailed help on this tool, call<a href="matlab:legacy_code('help')"> legacy_code('help')</a>.</p>
      mask Callback ShowSpec:
      | if strcmp(get_param(gcbh, 'ShowSpec'), 'on')
      |   set_param(gcbh, 'MaskDisplay', sprintf('fprintf(''%s'');', get_param(gcbh, 'SFunctionSpec')));
      | else
      |   set_param(gcbh, 'MaskDisplay', sprintf('fprintf(''%s'');', get_param(gcbh, 'FunctionName')));
      | end
      mask Display: fprintf('double y1 = pars_fcn(double u1, double u2, double u3, double u4, single u5)');
  "fault_id " : Constant  Value=3
  one : Constant
  corelation value : Outport
  wires:
  one/1 -> Discrete-Time Integrator/1
  Discrete-Time Integrator/1 -> ex_sfun_parsfcn/4, Scope1/2
  "fault_id "/1 -> ex_sfun_parsfcn/1
  SampleTime/1 -> ex_sfun_parsfcn/2
  SimLength/1 -> ex_sfun_parsfcn/3
  xml id/1 -> ex_sfun_parsfcn/5
  ex_sfun_parsfcn/1 -> Scope1/1, corelation value/1

== system SensorFaultInj/FIM_Muster1/Fault Injection Modul/MFI - multiplicative fault injection/time correlated noise/expr_parser1 ==
  xml id : Inport
  Discrete-Time Integrator : DiscreteIntegrator  SampleTime=-1  ICPrevOutput=DiscIntNeverNeededParam  ICPrevScaledInput=DiscIntNeverNeededParam
  SampleTime : Constant  Value=SampleTime
  Scope1 : Scope  NumInputPorts=2
      settings: YMin=-5~-5  YMax=5~5  SaveName=ScopeData24
  SimLength : Constant  Value=SimLength
  ex_sfun_parsfcn : S-Function  FunctionName=ex_sfun_parsfcn  EnableBusSupport=off  mask(Legacy Function){SFunctionSpec=double y1 = pars_fcn(double u1, double u2, double u3, double u4, single u5), ShowSpec=on}
      mask prompts: ShowSpec "Display function specification"
      mask help:
      | This block allows you to call the legacy functions specified by the following Legacy Code Tool definition:
      | def.SFunctionName = 'ex_sfun_parsfcn';
      | def.OutputFcnSpec = 'double y1 = pars_fcn(double u1, double u2, double u3, double u4, single u5)';
      | def.HeaderFiles = {'pars_fcn.hpp'};
      | def.SourceFiles = {'pars_fcn.cpp'};
      | def.Options.language = 'C++';
      mask Help: <p>This block was generated automatically by the Legacy Code Tool. For detailed help on this tool, call<a href="matlab:legacy_code('help')"> legacy_code('help')</a>.</p>
      mask Callback ShowSpec:
      | if strcmp(get_param(gcbh, 'ShowSpec'), 'on')
      |   set_param(gcbh, 'MaskDisplay', sprintf('fprintf(''%s'');', get_param(gcbh, 'SFunctionSpec')));
      | else
      |   set_param(gcbh, 'MaskDisplay', sprintf('fprintf(''%s'');', get_param(gcbh, 'FunctionName')));
      | end
      mask Display: fprintf('double y1 = pars_fcn(double u1, double u2, double u3, double u4, single u5)');
  "fault_id " : Constant  Value=2
  one : Constant
  corelation value : Outport
  wires:
  one/1 -> Discrete-Time Integrator/1
  Discrete-Time Integrator/1 -> ex_sfun_parsfcn/4, Scope1/2
  "fault_id "/1 -> ex_sfun_parsfcn/1
  SampleTime/1 -> ex_sfun_parsfcn/2
  SimLength/1 -> ex_sfun_parsfcn/3
  xml id/1 -> ex_sfun_parsfcn/5
  ex_sfun_parsfcn/1 -> Scope1/1, corelation value/1

== system SensorFaultInj/FIM_Muster1/Fault Injection Modul/MFI - multiplicative fault injection/time correlated noise/pdf_parser ==
  xml id : Inport
  Constant : Constant
  Interpreted MATLAB Function : MATLABFcn  MATLABFcn=rand
  Scope : Scope  NumInputPorts=2
      settings: YMin=0.05~2.77556e-17  YMax=0.85~1  SaveName=ScopeData26  MaxDataPoints=50000
  ex_sfun_parsdistr : S-Function  FunctionName=ex_sfun_parsdistr  EnableBusSupport=off  mask(Legacy Function){SFunctionSpec=double y1 = pars_distr(single u1, single u2, double u3), ShowSpec=on}
      mask prompts: ShowSpec "Display function specification"
      mask help:
      | This block allows you to call the legacy functions specified by the following Legacy Code Tool definition:
      | def.SFunctionName = 'ex_sfun_parsdistr';
      | def.OutputFcnSpec = 'double y1 = pars_distr(single u1, single u2, double u3)';
      | def.HeaderFiles = {'pars_distr.hpp'};
      | def.SourceFiles = {'pars_distr.cpp'};
      | def.Options.language = 'C++';
      mask Help: <p>This block was generated automatically by the Legacy Code Tool. For detailed help on this tool, call<a href="matlab:legacy_code('help')"> legacy_code('help')</a>.</p>
      mask Callback ShowSpec:
      | if strcmp(get_param(gcbh, 'ShowSpec'), 'on')
      |   set_param(gcbh, 'MaskDisplay', sprintf('fprintf(''%s'');', get_param(gcbh, 'SFunctionSpec')));
      | else
      |   set_param(gcbh, 'MaskDisplay', sprintf('fprintf(''%s'');', get_param(gcbh, 'FunctionName')));
      | end
      mask Display: fprintf('double y1 = pars_distr(single u1, single u2, double u3)');
  "fault_id " : Constant  Value=3  OutDataTypeStr=single
  distr value : Outport
  wires:
  "fault_id "/1 -> ex_sfun_parsdistr/1
  xml id/1 -> ex_sfun_parsdistr/2
  ex_sfun_parsdistr/1 -> Scope/1, distr value/1
  Constant/1 -> Interpreted MATLAB Function/1
  Interpreted MATLAB Function/1 -> ex_sfun_parsdistr/3, Scope/2

== system SensorFaultInj/FIM_Muster1/Fault Injection Modul/MFI - multiplicative fault injection/time correlated offset/expr_parser ==
  xml id : Inport
  Discrete-Time Integrator : DiscreteIntegrator  SampleTime=-1  ICPrevOutput=DiscIntNeverNeededParam  ICPrevScaledInput=DiscIntNeverNeededParam
  SampleTime : Constant  Value=SampleTime
  Scope1 : Scope  NumInputPorts=2
      settings: YMin=-5~-5  YMax=5~5  SaveName=ScopeData24
  SimLength : Constant  Value=SimLength
  ex_sfun_parsfcn : S-Function  FunctionName=ex_sfun_parsfcn  EnableBusSupport=off  mask(Legacy Function){SFunctionSpec=double y1 = pars_fcn(double u1, double u2, double u3, double u4, single u5), ShowSpec=on}
      mask prompts: ShowSpec "Display function specification"
      mask help:
      | This block allows you to call the legacy functions specified by the following Legacy Code Tool definition:
      | def.SFunctionName = 'ex_sfun_parsfcn';
      | def.OutputFcnSpec = 'double y1 = pars_fcn(double u1, double u2, double u3, double u4, single u5)';
      | def.HeaderFiles = {'pars_fcn.hpp'};
      | def.SourceFiles = {'pars_fcn.cpp'};
      | def.Options.language = 'C++';
      mask Help: <p>This block was generated automatically by the Legacy Code Tool. For detailed help on this tool, call<a href="matlab:legacy_code('help')"> legacy_code('help')</a>.</p>
      mask Callback ShowSpec:
      | if strcmp(get_param(gcbh, 'ShowSpec'), 'on')
      |   set_param(gcbh, 'MaskDisplay', sprintf('fprintf(''%s'');', get_param(gcbh, 'SFunctionSpec')));
      | else
      |   set_param(gcbh, 'MaskDisplay', sprintf('fprintf(''%s'');', get_param(gcbh, 'FunctionName')));
      | end
      mask Display: fprintf('double y1 = pars_fcn(double u1, double u2, double u3, double u4, single u5)');
  "fault_id " : Constant
  one : Constant
  corelation value : Outport
  wires:
  one/1 -> Discrete-Time Integrator/1
  Discrete-Time Integrator/1 -> ex_sfun_parsfcn/4, Scope1/2
  "fault_id "/1 -> ex_sfun_parsfcn/1
  SampleTime/1 -> ex_sfun_parsfcn/2
  SimLength/1 -> ex_sfun_parsfcn/3
  xml id/1 -> ex_sfun_parsfcn/5
  ex_sfun_parsfcn/1 -> Scope1/1, corelation value/1

== system SensorFaultInj/FIM_Muster1/Fault Injection Modul/MFI - multiplicative fault injection/value correlated noise/pdf_parser ==
  xml id : Inport
  Constant : Constant
  Interpreted MATLAB Function : MATLABFcn  MATLABFcn=rand
  Scope : Scope  NumInputPorts=2
      settings: YMin=0.05~2.77556e-17  YMax=0.85~1  SaveName=ScopeData26  MaxDataPoints=50000
  ex_sfun_parsdistr : S-Function  FunctionName=ex_sfun_parsdistr  EnableBusSupport=off  mask(Legacy Function){SFunctionSpec=double y1 = pars_distr(single u1, single u2, double u3), ShowSpec=on}
      mask prompts: ShowSpec "Display function specification"
      mask help:
      | This block allows you to call the legacy functions specified by the following Legacy Code Tool definition:
      | def.SFunctionName = 'ex_sfun_parsdistr';
      | def.OutputFcnSpec = 'double y1 = pars_distr(single u1, single u2, double u3)';
      | def.HeaderFiles = {'pars_distr.hpp'};
      | def.SourceFiles = {'pars_distr.cpp'};
      | def.Options.language = 'C++';
      mask Help: <p>This block was generated automatically by the Legacy Code Tool. For detailed help on this tool, call<a href="matlab:legacy_code('help')"> legacy_code('help')</a>.</p>
      mask Callback ShowSpec:
      | if strcmp(get_param(gcbh, 'ShowSpec'), 'on')
      |   set_param(gcbh, 'MaskDisplay', sprintf('fprintf(''%s'');', get_param(gcbh, 'SFunctionSpec')));
      | else
      |   set_param(gcbh, 'MaskDisplay', sprintf('fprintf(''%s'');', get_param(gcbh, 'FunctionName')));
      | end
      mask Display: fprintf('double y1 = pars_distr(single u1, single u2, double u3)');
  "fault_id " : Constant  Value=2  OutDataTypeStr=single
  distr value : Outport
  wires:
  "fault_id "/1 -> ex_sfun_parsdistr/1
  xml id/1 -> ex_sfun_parsdistr/2
  ex_sfun_parsdistr/1 -> Scope/1, distr value/1
  Constant/1 -> Interpreted MATLAB Function/1
  Interpreted MATLAB Function/1 -> ex_sfun_parsdistr/3, Scope/2
